simulink model "B_STUB"  (Simulink 8.1)
settings: Solver=ode1  StartTime=0.0  StopTime=1  FixedStep=Ts  MaxStep=1e-3  RelTol=1e-3
PostLoadFcn:
  | BANSHEE_init;
InitFcn:
  | BANSHEE_init;
values from neighbouring files (symbols this model uses):
  F2 = xlsread('F2_relay_banshee.xlsx')    [relay_settings_init.m]
  Ts = 100E-6    (= 0.0001)    [BANSHEE_init.m]
undefined symbols (not defined in the file or in its folder): cable_spec, Left, type, V
libraries: breaker_lib x20, relay_modbus_lib x19, rtio_generic_modbus x19, rtlab x18, cables_lib x11, transformer_lib x11, Load_lib x8, powerlib x6, ssn_lib x6, powerlib_extras x4, artemis x2, PQFV_lib x2
(part 2 of 2)

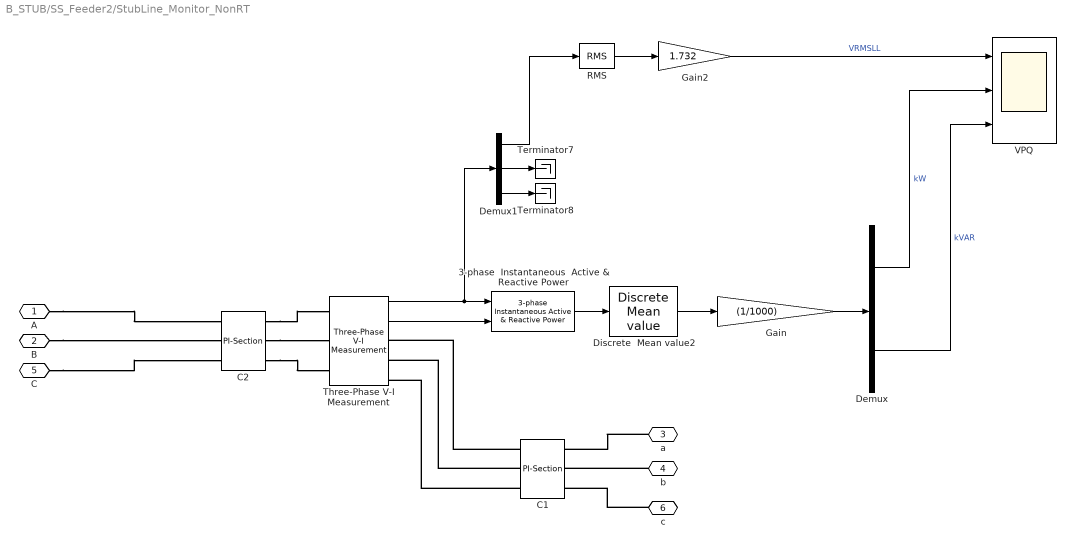
== system B_STUB/SS_Feeder2/StubLine_Monitor_NonRT ==
  3-phase  Instantaneous  Active & Reactive Power : powerlib_extras/Measurements/3-phase  Instantaneous  Active & Reactive Power
  C1 : cables_lib/PI-Section  cable_spec=[cable_spec(13, :)]  line_length=2500  parallel_sets=1
  C2 : cables_lib/PI-Section  cable_spec=[cable_spec(13, :)]  line_length=2500  parallel_sets=1
  Demux : Demux  Outputs=2
  Demux1 : Demux  Outputs=3
  Discrete  Mean value2 : powerlib_extras/Discrete Measurements/Discrete  Mean value  Freq=60  Vinit=0  Ts=Ts
  Gain : Gain  Gain=(1/1000)
  Gain2 : Gain  Gain=1.732
  RMS : PQFV_lib/PQFV/RMS
  Terminator7 : Terminator
  Terminator8 : Terminator
  Three-Phase V-I Measurement : powerlib/Measurements/Three-Phase V-I Measurement  VoltageMeasurement=phase-to-ground  SetLabelV=off  LabelV=Vabc  Vpu=off  VpuLL=off  CurrentMeasurement=yes  SetLabelI=off  LabelI=Iabc  Ipu=off  Pbase=100e6  Vbase=500e3  OutputType=Complex  PhasorSimulation=off  PSBequivalent=0
  VPQ : Scope  NumInputPorts=3
      settings: TimeRange=6  YMin=0~-500~-2100  YMax=15000~3750~0  SaveName=ScopeData2
  A : PMIOPort  Port=1  Side=Left
  B : PMIOPort  Port=2  Side=Left
  a : PMIOPort  Port=3  Side=Right
  b : PMIOPort  Port=4  Side=Right
  C : PMIOPort  Port=5  Side=Left
  c : PMIOPort  Port=6  Side=Right
  wires:
  Gain/1 -> Demux/1
  RMS/1 -> Gain2/1
  Demux1/3 -> Terminator8/1
  Demux1/2 -> Terminator7/1
  Demux1/1 -> RMS/1
  3-phase  Instantaneous  Active & Reactive Power/1 -> Discrete  Mean value2/1
  Discrete  Mean value2/1 -> Gain/1
  Three-Phase V-I Measurement/1 -> Demux1/1, 3-phase  Instantaneous  Active & Reactive Power/1
  Three-Phase V-I Measurement/2 -> 3-phase  Instantaneous  Active & Reactive Power/2
  Gain2/1 -> VPQ/1  "VRMSLL"
  Demux/1 -> VPQ/2  "kW"
  Demux/2 -> VPQ/3  "kVAR"
  connections:
  C/RConn1 -- C2/LConn3
  A/RConn1 -- C2/LConn1
  B/RConn1 -- C2/LConn2
  C2/RConn3 -- Three-Phase V-I Measurement/LConn3
  C2/RConn1 -- Three-Phase V-I Measurement/LConn1
  C2/RConn2 -- Three-Phase V-I Measurement/LConn2
  C1/LConn2 -- Three-Phase V-I Measurement/RConn2
  C1/LConn3 -- Three-Phase V-I Measurement/RConn3
  C1/LConn1 -- Three-Phase V-I Measurement/RConn1
  c/RConn1 -- C1/RConn3
  a/RConn1 -- C1/RConn1
  b/RConn1 -- C1/RConn2
